simulink model "pid_tuning_moo"  (R2025b)
settings: Solver=VariableStepAuto  StartTime=0.0  StopTime=T_end  RelTol=1e-3
undefined symbols (not defined in the file): A, B, C, D
libraries: slpidlib x1
settings Model: Creator=Ashraf AlAssi  LastModifiedBy=Ashraf AlAssi
settings RTWCC: GPUComputeCapability=3.5

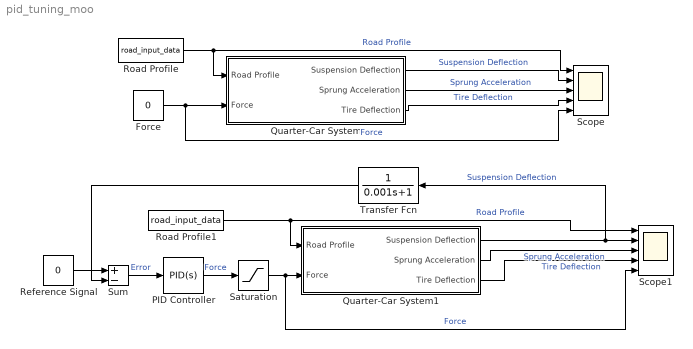
== system pid_tuning_moo ==
  Force : Constant  Value=0
  PID Controller : slpidlib/PID Controller  Controller=PID  Form=Parallel  TimeDomain=Continuous-time  UseExternalTs=off  SampleTime=-1  IntegratorMethod=Forward Euler  FilterMethod=Forward Euler  ControllerParametersSource=internal  P=19699.1514953811  I=159223.675591935  UseKiTs=off  D=315.685074639599  UseExternalDerivativeSource=off  N=1092.59450864332  UseFilter=on  TunerSelectOption=Transfer Function Based (PID Tuner App)  InitialConditionSource=internal  InitialConditionForIntegrator=0  InitialConditionForFilter=0  DifferentiatorICPrevScaledInput=0  ExternalReset=none  TrackingMode=off  Kt=1  LimitOutput=off  SatLimitsSource=internal  UpperSaturationLimit=inf  LowerSaturationLimit=-inf  LinearizeAsGain=on  AntiWindupMode=none  Kb=1  LimitIntegrator=off  UpperIntegratorSaturationLimit=inf  LowerIntegratorSaturationLimit=-inf  POutMin=[]  POutMax=[]  IOutMin=[]  IOutMax=[]  DOutMin=[]  DOutMax=[]  NOutMin=[]  NOutMax=[]  SumOutMin=[]  SumOutMax=[]  SaturationOutMin=[]  SaturationOutMax=[]  PParamMin=[]  PParamMax=[]  IParamMin=[]  IParamMax=[]  DParamMin=[]  DParamMax=[]  NParamMin=[]  NParamMax=[]  KbParamMin=[]  KbParamMax=[]  KtParamMin=[]  KtParamMax=[]  KbOutMin=[]  KbOutMax=[]  KtOutMin=[]  KtOutMax=[]  IntegratorOutMin=[]  IntegratorOutMax=[]  FilterOutMin=[]  FilterOutMax=[]  SumI1OutMin=[]  SumI1OutMax=[]  SumI2OutMin=[]  SumI2OutMax=[]  SumI3OutMin=[]  SumI3OutMax=[]  SumI4OutMin=[]  SumI4OutMax=[]  SumDOutMin=[]  SumDOutMax=[]  DifferentiatorOutMin=[]  DifferentiatorOutMax=[]  FilterDiffOutCoefMin=[]  FilterDiffOutCoefMax=[]  ReciprocalOutMin=[]  ReciprocalOutMax=[]  SumDenOutMin=[]  SumDenOutMax=[]  SumNumOutMin=[]  SumNumOutMax=[]  DivideOutMin=[]  DivideOutMax=[]  UdiffTsProdOutMin=[]  UdiffTsProdOutMax=[]  NTsProdOutMin=[]  NTsProdOutMax=[]  UintegralTsProdOutMin=[]  UintegralTsProdOutMax=[]  UngainTsProdOutMin=[]  UngainTsProdOutMax=[]  ClampingZeroOutDataTypeStr=Inherit: Inherit via back propagation  ClampingZeroOutMin=[]  ClampingZeroOutMax=[]  FilterDenConstantOutDataTypeStr=Inherit: Inherit via back propagation  FilterDenConstantOutMin=[]  FilterDenConstantOutMax=[]  PCopyOutDataTypeStr=Inherit: Inherit via back propagation  PCopyOutMin=[]  PCopyOutMax=[]  NCopyOutDataTypeStr=Inherit: Inherit via back propagation  NCopyOutMin=[]  NCopyOutMax=[]  IntegratorContinuousStateAttributes=''  IntegratorStateMustResolveToSignalObject=off  IntegratorRTWStateStorageClass=Auto  FilterContinuousStateAttributes=''  FilterStateMustResolveToSignalObject=off  FilterRTWStateStorageClass=Auto  ParallelPVariant=InternalParameters  IdealPVariant=Disabled  IVariant=InternalParameters  DVariant=InternalParameters  IntegratorVariant=Continuous  SatVariant=Disabled  AWVariant=Passthrough  PCopyVariant=Disabled  TRVariant=Disabled  FdbkBlocksVariant=Forward  IdealPFdbkVariant=Disabled  SatFdbkVariant=Disabled  DerivativeFilterVariant=ContFilter  NVariant=InternalParameters  NCopyVariant=Disabled  FilterICVariant=InternalICsFilter  IntegratorICVariant=InternalICs  ExternalResetVariant=Disabled  TRSumVariant=Passthrough  SumFdbkVariant=Disabled  SumVariant=Sum_PID  TsampFilterVariant=InternalTs  TsampNgainVariant=Passthrough  TsampIntegralVariant=Disabled_SignalSpec  ExternalSaturationOutDataTypeStr=Inherit: Same as second input  DerivativeSourceVariant=ErrorSignal  PreIntVariant=InternalPreInt
  Quarter-Car System : Subsystem
  Quarter-Car System1 : Subsystem
  Reference Signal : Constant  Value=0
  Road Profile : FromWorkspace  VariableName=road_input_data  OutputAfterFinalValue=Setting to zero
  Road Profile1 : FromWorkspace  VariableName=road_input_data  OutputAfterFinalValue=Setting to zero
  Saturation : Saturate  UpperLimit=+3000  LowerLimit=-3000
  Scope : Scope  NumInputPorts=5
      settings: SampleTime=0.0001  ActiveDisplayYMinimum=-43.62216  ActiveDisplayYMaximum=34.38842
  Scope1 : Scope  NumInputPorts=5
      settings: SampleTime=0.0001  ActiveDisplayYMinimum=-1.2500000000000004  ActiveDisplayYMaximum=1.25
  Sum : Sum  Inputs=+-
  Transfer Fcn : TransferFcn  Denominator=[0.001 1]
  wires:
  Force/1 -> Scope/5, Quarter-Car System/2(Force)  "Force"
  Road Profile/1 -> Quarter-Car System/1(Road Profile), Scope/1  "Road Profile"
  Quarter-Car System/1(Suspension Deflection) -> Scope/2  "Suspension Deflection"
  Quarter-Car System/2(Sprung Acceleration) -> Scope/3  "Sprung Acceleration"
  Quarter-Car System/3(Tire Deflection) -> Scope/4  "Tire Deflection"
  Quarter-Car System1/1(Suspension Deflection) -> Transfer Fcn/1, Scope1/2  "Suspension Deflection"
  PID Controller/1 -> Saturation/1  "Force"
  Road Profile1/1 -> Scope1/1, Quarter-Car System1/1(Road Profile)  "Road Profile"
  Quarter-Car System1/3(Tire Deflection) -> Scope1/4  "Tire Deflection"
  Quarter-Car System1/2(Sprung Acceleration) -> Scope1/3  "Sprung Acceleration"
  Reference Signal/1 -> Sum/1
  Sum/1 -> PID Controller/1  "Error"
  Saturation/1 -> Scope1/5, Quarter-Car System1/2(Force)  "Force"
  Transfer Fcn/1 -> Sum/2

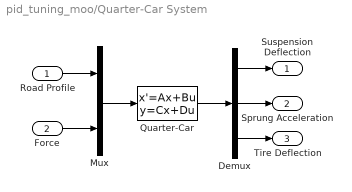
== system pid_tuning_moo/Quarter-Car System ==
  Road Profile : Inport
  Force : Inport  Port=2
  Demux : Demux  Outputs=3
  Mux : Mux  Inputs=2
  Quarter-Car : StateSpace  A=A  B=B  C=C  D=D  InitialCondition=[0; 0; 0; 0]
  Suspension Deflection : Outport
  Sprung Acceleration : Outport  Port=2
  Tire Deflection : Outport  Port=3
  wires:
  Mux/1 -> Quarter-Car/1
  Quarter-Car/1 -> Demux/1
  Demux/3 -> Tire Deflection/1
  Road Profile/1 -> Mux/1
  Demux/1 -> Suspension Deflection/1
  Demux/2 -> Sprung Acceleration/1
  Force/1 -> Mux/2

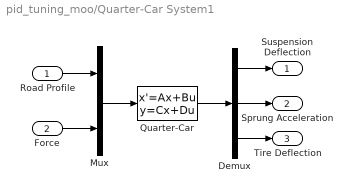
== system pid_tuning_moo/Quarter-Car System1 ==
  Road Profile : Inport
  Force : Inport  Port=2
  Demux : Demux  Outputs=3
  Mux : Mux  Inputs=2
  Quarter-Car : StateSpace  A=A  B=B  C=C  D=D  InitialCondition=[0; 0; 0; 0]
  Suspension Deflection : Outport
  Sprung Acceleration : Outport  Port=2
  Tire Deflection : Outport  Port=3
  wires:
  Mux/1 -> Quarter-Car/1
  Quarter-Car/1 -> Demux/1
  Demux/3 -> Tire Deflection/1
  Road Profile/1 -> Mux/1
  Demux/1 -> Suspension Deflection/1
  Demux/2 -> Sprung Acceleration/1
  Force/1 -> Mux/2
